simulink model "ThreecellsSolarArrayWithSprings_damp"  (R2016a)
settings: Solver=VariableStepAuto  StartTime=0.0  StopTime=10.0  RelTol=1e-3
values from neighbouring files (symbols this model uses):
  C = 1    [Copy_of_example_3pannels.m]    (also in example_3pannels.m)
  K = 1e2    (= 100)    [Copy_of_example_3pannels.m]    (also in example_3pannels.m)
libraries: cstblocks x3
settings Model: Creator=f.sanfedino  LastModifiedBy=f.sanfedino

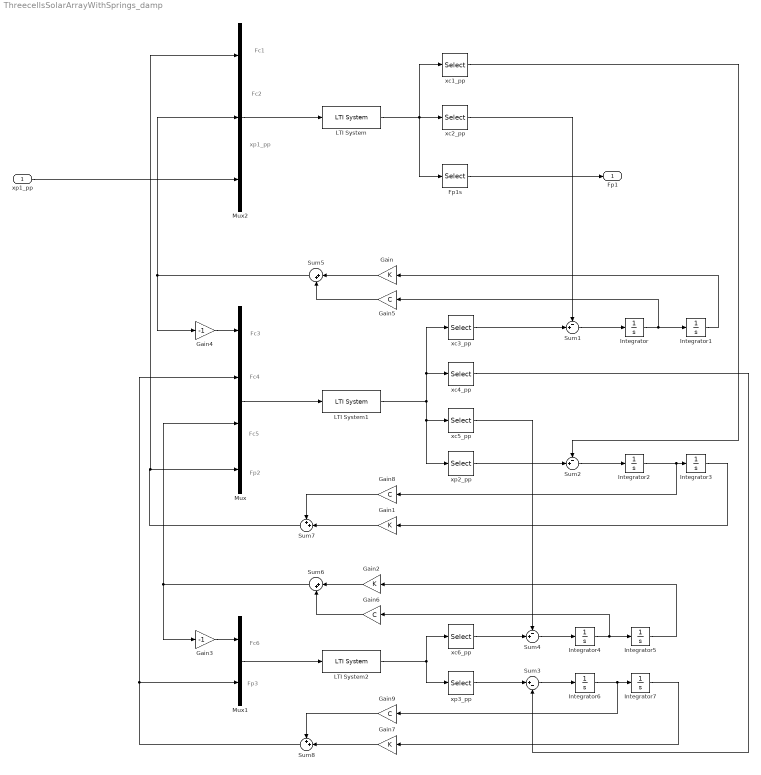
== system ThreecellsSolarArrayWithSprings_damp ==
  note: Fc6
  note: xp1_pp
  note: Fc2
  note: Fc1
  note: Fp2
  note: Fc5
  note: Fc4
  note: Fc3
  note: Fp3
  xp1_pp : Inport  PortDimensions=3
  Fp1s : Selector  InputPortWidth=9  IndexOptions=Index vector (dialog)  Indices=[7:9]  OutputSizes=1
  Gain{,1..2,7} (4 alike) : Gain  Gain=K
  Gain3 : Gain  Gain=-1
  Gain4 : Gain  Gain=-1
  Gain{5..6,8..9} (4 alike) : Gain  Gain=C
  Integrator{,1..7} (8 alike) : Integrator
  LTI System : cstblocks/LTI System  sys=M1  IC=[]
  LTI System1 : cstblocks/LTI System  sys=M2_inv2  IC=[]
  LTI System2 : cstblocks/LTI System  sys=M3_inv2  IC=[]
  Mux : Mux
  Mux1 : Mux  Inputs=2
  Mux2 : Mux  Inputs=3
  Sum1 : Sum  Inputs=-+|
  Sum2 : Sum  Inputs=-+|
  Sum3 : Sum  Inputs=|+-
  Sum4 : Sum  Inputs=-+|
  Sum5 : Sum  Inputs=|++
  Sum6 : Sum  Inputs=|++
  Sum7 : Sum  Inputs=++|
  Sum8 : Sum  Inputs=++|
  xc1_pp : Selector  InputPortWidth=9  IndexOptions=Index vector (dialog)  Indices=[1:3]  OutputSizes=1
  xc2_pp : Selector  InputPortWidth=9  IndexOptions=Index vector (dialog)  Indices=[4:6]  OutputSizes=1
  xc3_pp : Selector  InputPortWidth=12  IndexOptions=Index vector (dialog)  Indices=[1:3]  OutputSizes=1
  xc4_pp : Selector  InputPortWidth=12  IndexOptions=Index vector (dialog)  Indices=[4:6]  OutputSizes=1
  xc5_pp : Selector  InputPortWidth=12  IndexOptions=Index vector (dialog)  Indices=[7:9]  OutputSizes=1
  xc6_pp : Selector  InputPortWidth=6  IndexOptions=Index vector (dialog)  Indices=[1:3]  OutputSizes=1
  xp2_pp : Selector  InputPortWidth=12  IndexOptions=Index vector (dialog)  Indices=[10:12]  OutputSizes=1
  xp3_pp : Selector  InputPortWidth=6  IndexOptions=Index vector (dialog)  Indices=[4:6]  OutputSizes=1
  Fp1 : Outport
  wires:
  LTI System/1 -> Fp1s/1, xc2_pp/1, xc1_pp/1
  LTI System1/1 -> xc5_pp/1, xp2_pp/1, xc3_pp/1, xc4_pp/1
  LTI System2/1 -> xp3_pp/1, xc6_pp/1
  Mux2/1 -> LTI System/1
  Mux/1 -> LTI System1/1
  Mux1/1 -> LTI System2/1
  xc1_pp/1 -> Sum2/1
  xp1_pp/1 -> Mux2/3
  Fp1s/1 -> Fp1/1
  Integrator/1 -> Gain5/1, Integrator1/1
  xc3_pp/1 -> Sum1/2
  xc2_pp/1 -> Sum1/1
  Sum1/1 -> Integrator/1
  Integrator1/1 -> Gain/1
  Sum2/1 -> Integrator2/1
  Integrator2/1 -> Gain8/1, Integrator3/1
  Integrator3/1 -> Gain1/1
  xc6_pp/1 -> Sum4/2
  Sum4/1 -> Integrator4/1
  Integrator4/1 -> Gain6/1, Integrator5/1
  Integrator5/1 -> Gain2/1
  Sum3/1 -> Integrator6/1
  Integrator6/1 -> Gain9/1, Integrator7/1
  Integrator7/1 -> Gain7/1
  xc5_pp/1 -> Sum4/1
  xc4_pp/1 -> Sum3/2
  xp2_pp/1 -> Sum2/2
  xp3_pp/1 -> Sum3/1
  Gain3/1 -> Mux1/1
  Gain4/1 -> Mux/1
  Gain/1 -> Sum5/1
  Sum5/1 -> Gain4/1, Mux2/2
  Gain5/1 -> Sum5/2
  Gain2/1 -> Sum6/1
  Sum6/1 -> Gain3/1, Mux/3
  Gain6/1 -> Sum6/2
  Gain1/1 -> Sum7/2
  Sum7/1 -> Mux2/1, Mux/4
  Gain8/1 -> Sum7/1
  Gain7/1 -> Sum8/2
  Sum8/1 -> Mux/2, Mux1/2
  Gain9/1 -> Sum8/1
